simulink model "Cascade_Function"  (R2020a)
settings: Solver=FixedStepAuto  StartTime=0.0  StopTime=10.0  FixedStep=0.2  RelTol=1e-3
settings Model: Creator=Atri Mondal  LastModifiedBy=Atri Mondal
settings DataIOCC: SaveOutput=off  SaveTime=off

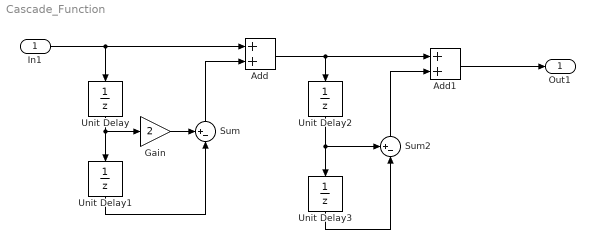
== system Cascade_Function ==
  In1 : Inport  OutDataTypeStr=double  PortDimensions=1  SampleTime=[0.20000000000000001,0]
  Add : Sum
  Add1 : Sum
  Gain : Gain  Gain=2
  Sum : Sum  Inputs=+-|
  Sum2 : Sum  Inputs=+-|
  Unit Delay{,1..3} (4 alike) : UnitDelay  SampleTime=-1  HasFrameUpgradeWarning=on
  Out1 : Outport  OutDataTypeStr=double  PortDimensions=1  SampleTime=[0.20000000000000001,0]
  wires:
  Sum2/1 -> Add1/2
  Sum/1 -> Add/2
  In1/1 -> Add/1, Unit Delay/1
  Unit Delay2/1 -> Unit Delay3/1, Sum2/1
  Unit Delay1/1 -> Sum/2
  Unit Delay/1 -> Unit Delay1/1, Gain/1
  Unit Delay3/1 -> Sum2/2
  Add/1 -> Unit Delay2/1, Add1/1
  Gain/1 -> Sum/1
  Add1/1 -> Out1/1
